simulink model "sampleModel1875"  (R2023a)
settings: Solver=VariableStepAuto  StartTime=0.0  StopTime=10.0  RelTol=1e-3
libraries: hdlsllib x2, simulink x1
settings Model: Creator=user1  LastModifiedBy=user1

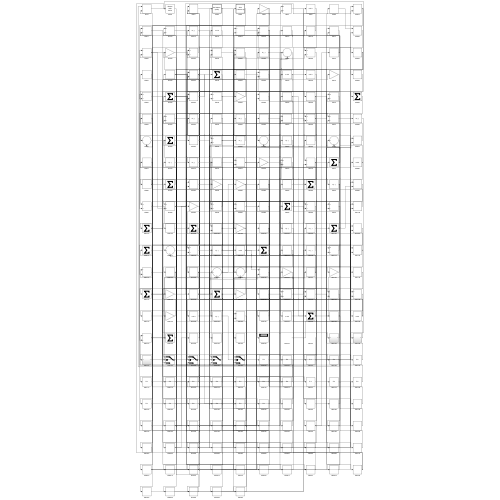
[thumbnail: Simulink's stored preview of the top-level diagram]
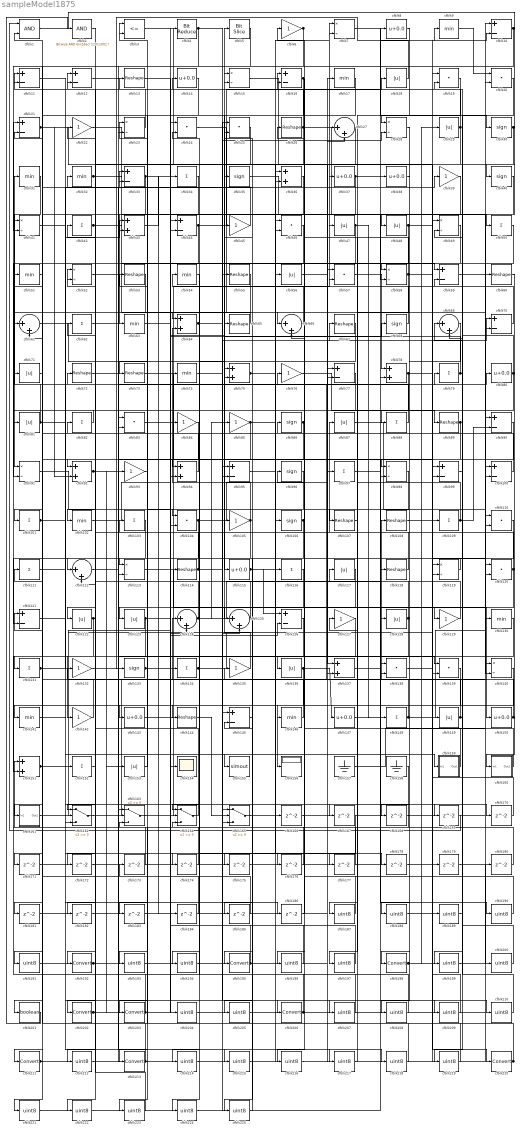
== system sampleModel1875 ==
  cfblk1 : Logic  AllPortsSameDT=off  OutDataTypeStr=boolean
  cfblk{10..12,16,21,33,44,59,70,77,90,95,99..100,121,126,145} (17 alike) : Sum  Inputs=+-
  cfblk{34,42,50,62,79,82,88,97,101,103,109,111,116,131,134,148,152} (17 alike) : Sum  Inputs=+
  cfblk{9,17,31..32,51,54,63,74,102,130,141,146} (12 alike) : MinMax
  cfblk{19..20,24..25,46,57,83,104,110,120,138..139} (12 alike) : DotProduct  OutDataTypeStr=Inherit: Inherit via internal rule
  cfblk{6,22,39,45,76,84..85,93,105,127,129,132,135,142} (14 alike) : Gain
  cfblk{30,35,40,68,86,96,106,133} (8 alike) : Signum
  cfblk{13,26,53,55,60,65,67,72..73,89,107..108,114,118,144} (15 alike) : Reshape
  cfblk{27,61,66,69,112,124..125} (7 alike) : Sum  Inputs=|++
  cfblk{7,15,23,28,41,49,52,58,91,98,113,119,140} (13 alike) : Product  Inputs=*/  RndMeth=Zero  SaturateOnIntegerOverflow=on
  cfblk{8,14,37..38,80,115,143,147,150} (9 alike) : Bias  Bias=0.0  SaturateOnIntegerOverflow=off
  cfblk{18,29,47..48,56,71,81,87,117,122..123,128,136,149,153} (15 alike) : Abs  SaturateOnIntegerOverflow=off
  cfblk{36,43,64,75,78,92,94,137,151} (9 alike) : Sum
  cfblk154 : Scope
  cfblk155 : ToWorkspace  VariableName=simout  SaveFormat=Timeseries  SampleTime=-1
  cfblk156 : Display
  cfblk157 : Ground
  cfblk158 : Ground
  cfblk159 : Subsystem
      settings: LibrarySourceBlock=|
      | hdlsllib/Ports &
      | Subsystems/Subsystem
  cfblk160 : Subsystem
      settings: LibrarySourceBlock=|
      | hdlsllib/Ports &
      | Subsystems/Subsystem
  cfblk161 : Subsystem
      settings: LibrarySourceBlock=|
      | hdlsllib/Ports &
      | Subsystems/Subsystem
  cfblk{162..165} (4 alike) : Switch  SaturateOnIntegerOverflow=off  InputSameDT=off
  cfblk{166..186} (21 alike) : Delay  SampleTime=1
  cfblk{187..191,193..194,196..197,199..200,204..205,207..210,212,214..219,221..225} (29 alike) : DataTypeConversion  OutDataTypeStr=uint8  SaturateOnIntegerOverflow=off  RndMeth=Floor
  cfblk{192,195,198,202..203,206,211,213,220} (9 alike) : DataTypeConversion  SaturateOnIntegerOverflow=off  RndMeth=Floor
  cfblk2 : simulink/Logic and Bit Operations/Bitwise Operator  logicop=AND  UseBitMask=on  BitMask=bin2dec('11011001')  BitMaskRealWorld=Stored Integer
      settings: LibrarySourceBlock=|
      | hdlsllib/Logic and Bit
      | Operations/Bitwise
      | Operator
  cfblk201 : DataTypeConversion  OutDataTypeStr=boolean  SaturateOnIntegerOverflow=off  RndMeth=Floor
  cfblk3 : RelationalOperator  Operator=<=  OutDataTypeStr=boolean  InputSameDT=off
  cfblk4 : hdlsllib/Logic and Bit Operations/Bit Reduce  mode=AND
  cfblk5 : hdlsllib/Logic and Bit Operations/Bit Slice  lidx=7  ridx=0
  wires:
  cfblk135/1 -> cfblk5/1
  cfblk120/1 -> cfblk87/1, cfblk163/2
  cfblk161/1(Out1) -> cfblk79/1
  cfblk158/1 -> cfblk151/1
  cfblk66/1 -> cfblk54/1
  cfblk31/1 -> cfblk91/1
  cfblk43/1 -> cfblk34/1
  cfblk138/1 -> cfblk220/1
  cfblk153/1 -> cfblk23/1
  cfblk143/1 -> cfblk7/1
  cfblk18/1 -> cfblk133/1
  cfblk85/1 -> cfblk99/2, cfblk214/1
  cfblk51/1 -> cfblk131/1
  cfblk17/1 -> cfblk115/1
  cfblk162/1 -> cfblk108/1
  cfblk75/1 -> cfblk7/2, cfblk177/1
  cfblk136/1 -> cfblk147/1, cfblk185/1
  cfblk124/1 -> cfblk38/1, cfblk53/1, cfblk85/1
  cfblk61/1 -> cfblk75/1
  cfblk81/1 -> cfblk31/1, cfblk43/1
  cfblk48/1 -> cfblk91/2, cfblk120/2
  cfblk149/1 -> cfblk124/1, cfblk219/1
  cfblk44/1 -> cfblk18/1, cfblk92/1
  cfblk14/1 -> cfblk73/1
  cfblk89/1 -> cfblk136/1, cfblk188/1
  cfblk65/1 -> cfblk64/1
  cfblk159/1(Out1) -> cfblk76/1
  cfblk113/1 -> cfblk150/1
  cfblk1/1 -> cfblk40/1
  cfblk106/1 -> cfblk171/1, cfblk221/1, cfblk225/1
  cfblk105/1 -> cfblk64/2, cfblk164/2
  cfblk100/1 -> cfblk82/1
  cfblk82/1 -> cfblk81/1
  cfblk83/1 -> cfblk44/2
  cfblk36/1 -> cfblk213/1
  cfblk9/1 -> cfblk20/1
  cfblk35/1 -> cfblk48/1
  cfblk69/1 -> cfblk198/1
  cfblk39/1 -> cfblk63/1
  cfblk123/1 -> cfblk134/1, cfblk222/1
  cfblk116/1 -> cfblk125/1
  cfblk118/1 -> cfblk32/1
  cfblk109/1 -> cfblk47/1, cfblk90/2
  cfblk10/1 -> cfblk50/1, cfblk41/2
  cfblk84/1 -> cfblk141/1
  cfblk139/1 -> cfblk161/1(In1)
  cfblk4/1 -> cfblk61/1, cfblk98/2
  cfblk79/1 -> cfblk15/1, cfblk59/2
  cfblk163/1 -> cfblk60/1
  cfblk59/1 -> cfblk20/2
  cfblk76/1 -> cfblk89/1
  cfblk134/1 -> cfblk99/1, cfblk224/1
  cfblk99/1 -> cfblk129/1
  cfblk21/1 -> cfblk119/2, cfblk92/2
  cfblk128/1 -> cfblk72/1, cfblk75/2, cfblk162/2
  cfblk53/1 -> cfblk122/1
  cfblk157/1 -> cfblk120/1
  cfblk145/1 -> cfblk195/1
  cfblk13/1 -> cfblk114/1
  cfblk96/1 -> cfblk104/1
  cfblk148/1 -> cfblk90/1, cfblk62/1
  cfblk2/1 -> cfblk202/1
  cfblk30/1 -> cfblk102/1, cfblk162/1
  cfblk151/1 -> cfblk128/1, cfblk186/1
  cfblk140/1 -> cfblk156/1
  cfblk146/1 -> cfblk13/1
  cfblk57/1 -> cfblk78/1
  cfblk87/1 -> cfblk140/1
  cfblk115/1 -> cfblk116/1, cfblk126/1
  cfblk74/1 -> cfblk206/1
  cfblk50/1 -> cfblk88/1
  cfblk114/1 -> cfblk159/1(In1), cfblk70/1, cfblk33/1
  cfblk86/1 -> cfblk104/2, cfblk172/1
  cfblk119/1 -> cfblk113/1
  cfblk122/1 -> cfblk142/1, cfblk52/2
  cfblk33/1 -> cfblk184/1, cfblk201/1
  cfblk45/1 -> cfblk21/2
  cfblk8/1 -> cfblk28/1
  cfblk110/1 -> cfblk203/1
  cfblk129/1 -> cfblk3/1
  cfblk90/1 -> cfblk144/1
  cfblk130/1 -> cfblk151/2
  cfblk29/1 -> cfblk3/2, cfblk16/1, cfblk94/2
  cfblk150/1 -> cfblk135/1, cfblk103/1
  cfblk26/1 -> cfblk130/1, cfblk14/1, cfblk165/3
  cfblk15/1 -> cfblk137/1
  cfblk60/1 -> cfblk160/1(In1)
  cfblk88/1 -> cfblk51/1
  cfblk73/1 -> cfblk95/2
  cfblk24/1 -> cfblk66/1
  cfblk5/1 -> cfblk101/1
  cfblk152/1 -> cfblk22/1
  cfblk42/1 -> cfblk109/1, cfblk77/2, cfblk175/1
  cfblk37/1 -> cfblk9/1, cfblk162/3
  cfblk41/1 -> cfblk152/1
  cfblk131/1 -> cfblk68/1, cfblk33/2
  cfblk147/1 -> cfblk8/1
  cfblk6/1 -> cfblk113/2, cfblk23/2
  cfblk55/1 -> cfblk211/1
  cfblk98/1 -> cfblk143/1
  cfblk92/1 -> cfblk98/1, cfblk39/1
  cfblk125/1 -> cfblk35/1, cfblk52/1, cfblk105/1
  cfblk144/1 -> cfblk165/2
  cfblk7/1 -> cfblk30/1
  cfblk72/1 -> cfblk139/1
  cfblk121/1 -> cfblk155/1
  cfblk38/1 -> cfblk58/1
  cfblk32/1 -> cfblk149/1, cfblk58/2, cfblk217/1
  cfblk142/1 -> cfblk121/1
  cfblk133/1 -> cfblk65/1, cfblk126/2
  cfblk54/1 -> cfblk94/1
  cfblk58/1 -> cfblk107/1, cfblk10/2, cfblk16/2
  cfblk80/1 -> cfblk15/2, cfblk146/1
  cfblk23/1 -> cfblk11/1
  cfblk52/1 -> cfblk140/2
  cfblk160/1(Out1) -> cfblk57/2
  cfblk164/1 -> cfblk12/1
  cfblk101/1 -> cfblk37/1, cfblk207/1
  cfblk117/1 -> cfblk123/1
  cfblk104/1 -> cfblk121/2, cfblk24/2, cfblk27/2
  cfblk47/1 -> cfblk66/2, cfblk148/1
  cfblk112/1 -> cfblk80/1
  cfblk137/1 -> cfblk118/1
  cfblk91/1 -> cfblk154/1
  cfblk16/1 -> cfblk61/2, cfblk176/1
  cfblk64/1 -> cfblk28/2, cfblk169/1
  cfblk56/1 -> cfblk139/2
  cfblk67/1 -> cfblk164/1
  cfblk3/1 -> cfblk106/1
  cfblk46/1 -> cfblk192/1
  cfblk78/1 -> cfblk112/1, cfblk70/2
  cfblk70/1 -> cfblk6/1
  cfblk102/1 -> cfblk84/1
  cfblk95/1 -> cfblk67/1
  cfblk68/1 -> cfblk45/1
  cfblk94/1 -> cfblk11/2
  cfblk22/1 -> cfblk59/1
  cfblk166/1 -> cfblk100/2
  cfblk11/1 -> cfblk167/1
  cfblk28/1 -> cfblk168/1
  cfblk168/1 -> cfblk10/1
  cfblk169/1 -> cfblk1/1
  cfblk165/1 -> cfblk170/1
  cfblk170/1 -> cfblk119/1
  cfblk171/1 -> cfblk57/1
  cfblk172/1 -> cfblk43/2
  cfblk173/1 -> cfblk112/2
  cfblk62/1 -> cfblk174/1
  cfblk174/1 -> cfblk21/1
  cfblk175/1 -> cfblk78/2
  cfblk176/1 -> cfblk12/2
  cfblk177/1 -> cfblk44/1
  cfblk141/1 -> cfblk178/1
  cfblk108/1 -> cfblk179/1
  cfblk180/1 -> cfblk164/3
  cfblk71/1 -> cfblk181/1
  cfblk181/1 -> cfblk163/1
  cfblk103/1 -> cfblk182/1
  cfblk182/1 -> cfblk125/2
  cfblk93/1 -> cfblk183/1
  cfblk183/1 -> cfblk137/2
  cfblk184/1 -> cfblk163/3
  cfblk185/1 -> cfblk1/2
  cfblk186/1 -> cfblk26/1
  cfblk19/1 -> cfblk187/1
  cfblk187/1 -> cfblk96/1
  cfblk188/1 -> cfblk19/1
  cfblk189/1 -> cfblk19/2
  cfblk97/1 -> cfblk190/1
  cfblk190/1 -> cfblk86/1
  cfblk77/1 -> cfblk191/1
  cfblk191/1 -> cfblk97/1
  cfblk192/1 -> cfblk27/1, cfblk153/1, cfblk124/2
  cfblk34/1 -> cfblk193/1
  cfblk193/1 -> cfblk46/1
  cfblk167/1 -> cfblk194/1
  cfblk194/1 -> cfblk46/2
  cfblk195/1 -> cfblk166/1, cfblk24/1
  cfblk27/1 -> cfblk196/1
  cfblk196/1 -> cfblk145/1
  cfblk107/1 -> cfblk197/1
  cfblk197/1 -> cfblk145/2
  cfblk198/1 -> cfblk180/1, cfblk29/1
  cfblk20/1 -> cfblk199/1
  cfblk199/1 -> cfblk69/1
  cfblk179/1 -> cfblk200/1
  cfblk200/1 -> cfblk69/2
  cfblk201/1 -> cfblk2/1
  cfblk202/1 -> cfblk4/1, cfblk93/1
  cfblk203/1 -> cfblk41/1, cfblk165/1
  cfblk63/1 -> cfblk204/1
  cfblk204/1 -> cfblk110/1
  cfblk126/1 -> cfblk205/1
  cfblk205/1 -> cfblk110/2
  cfblk206/1 -> cfblk111/1, cfblk95/1
  cfblk207/1 -> cfblk74/1
  cfblk49/1 -> cfblk208/1
  cfblk208/1 -> cfblk83/1
  cfblk12/1 -> cfblk209/1
  cfblk209/1 -> cfblk49/1
  cfblk178/1 -> cfblk210/1
  cfblk210/1 -> cfblk49/2
  cfblk211/1 -> cfblk83/2, cfblk56/1, cfblk17/1
  cfblk40/1 -> cfblk212/1
  cfblk212/1 -> cfblk55/1
  cfblk213/1 -> cfblk189/1, cfblk71/1
  cfblk214/1 -> cfblk36/1
  cfblk111/1 -> cfblk215/1
  cfblk215/1 -> cfblk36/2
  cfblk127/1 -> cfblk216/1
  cfblk216/1 -> cfblk100/1
  cfblk217/1 -> cfblk127/1
  cfblk132/1 -> cfblk218/1
  cfblk218/1 -> cfblk117/1
  cfblk219/1 -> cfblk132/1
  cfblk220/1 -> cfblk173/1, cfblk77/1
  cfblk221/1 -> cfblk138/1
  cfblk222/1 -> cfblk138/2
  cfblk25/1 -> cfblk223/1
  cfblk223/1 -> cfblk42/1
  cfblk224/1 -> cfblk25/1
  cfblk225/1 -> cfblk25/2

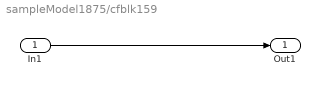
== system sampleModel1875/cfblk159 ==
  In1 : Inport
  Out1 : Outport
  wires:
  In1/1 -> Out1/1

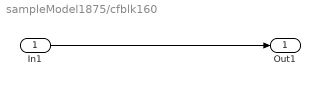
== system sampleModel1875/cfblk160 ==
  In1 : Inport
  Out1 : Outport
  wires:
  In1/1 -> Out1/1

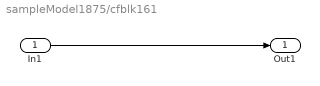
== system sampleModel1875/cfblk161 ==
  In1 : Inport
  Out1 : Outport
  wires:
  In1/1 -> Out1/1
